simulink model "pservop1"  (Simulink 3.00)
settings: Solver=ode45  StartTime=0.0  StopTime=999999  MaxStep=10  RelTol=1e-3  AbsTol=1e-3
values from neighbouring files (symbols this model uses):
  A1 = 19.63e-4    (= 0.001963)    [pservpar.m]
  A2 = 16.49e-4    (= 0.001649)    [pservpar.m]
  B1 = 30    [pservpar.m]
  Fdry = 0    [pservpar.m]
  g = 9.81    [pservpar.m]
  k1 = 1.4    [pservpar.m]
  kkrit = 1.3154    [pservpar.m]
  kvalve = 2.857e-9    (= 2.857e-09)    [pservpar.m]
  M = 20.    (= 20)    [pservpar.m]
  P10 = 4.e5    (= 400000)    [pservpar.m]
  P20 = (M*g+P10*A1-PR*(A1-A2))/A2    (= 576106.731352)    [pservpar.m]
  PR = 1e5    (= 100000)    [pservpar.m]
  PS = 6e5    (= 600000)    [pservpar.m]
  R1 = 281.3    [pservpar.m]
  rho1 = 1.208    [pservpar.m]
  T1 = 293    [pservpar.m]
  V1 = 4.908e-4    (= 0.0004908)    [pservpar.m]
  V2 = 4.123e-4    (= 0.0004123)    [pservpar.m]
  X0 = 0    [pservpar.m]
  zkrit = 0.528    [pservpar.m]
settings Model: SaveTime=off  SaveOutput=off  Creator=pmn  LastModifiedBy=pmn

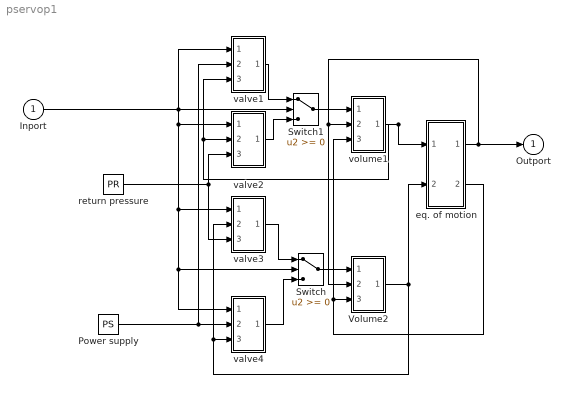
== system pservop1 ==
  Inport : Inport  Port=1  PortWidth=-1  SampleTime=-1  DataType=auto
      settings: SignalType=auto
  Power supply : Constant  Value=PS
  Switch : Switch  Threshold=0
  Switch1 : Switch  Threshold=0
  Volume2 : Subsystem
  eq. of motion : Subsystem
  return pressure : Constant  Value=PR
  valve1 : Subsystem
  valve2 : Subsystem
  valve3 : Subsystem
  valve4 : Subsystem
  volume1 : Subsystem
  Outport : Outport  Port=1
  wires:
  valve3/1(out_1) -> Switch/1
  valve1/1(out_1) -> Switch1/1
  Power supply/1 -> valve4/2(in_2), valve1/2(in_2)
  Inport/1 -> Switch1/2, valve4/1(in_1), Switch/2, valve3/1(in_1), valve2/1(in_1), valve1/1(in_1)
  valve2/1(out_1) -> Switch1/3
  valve4/1(out_1) -> Switch/3
  return pressure/1 -> valve2/3(in_3), valve3/3(in_3)
  volume1/1(out_1) -> eq. of motion/1(in_1), valve2/2(in_2), valve1/3(in_3)
  Switch1/1 -> volume1/1(in_1)
  Switch/1 -> Volume2/1(in_1)
  eq. of motion/1(position) -> Outport/1, Volume2/2(in_2), volume1/2(in_2)
  eq. of motion/2(velocity) -> volume1/3(in_3), Volume2/3(in_3)
  Volume2/1(out_1) -> eq. of motion/2(in_2), valve3/2(in_2), valve4/3(in_3)

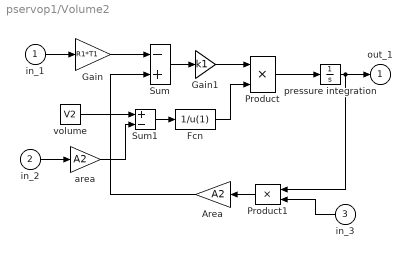
== system pservop1/Volume2 ==
  in_1 : Inport  Port=1  PortWidth=-1  SampleTime=-1  DataType=auto
      settings: SignalType=auto
  in_2 : Inport  Port=2  PortWidth=-1  SampleTime=-1  DataType=auto
      settings: SignalType=auto
  in_3 : Inport  Orientation=left  Port=3  PortWidth=-1  SampleTime=-1  DataType=auto
      settings: SignalType=auto
  Area : Gain  Orientation=left  Gain=A2  SaturateOnIntegerOverflow=on
  Fcn : Fcn  Expr=1/u(1)
  Gain : Gain  Gain=R1*T1  SaturateOnIntegerOverflow=on
  Gain1 : Gain  Gain=k1  SaturateOnIntegerOverflow=on
  Product : Product  Inputs=2  SaturateOnIntegerOverflow=on
  Product1 : Product  Orientation=left  Inputs=2  SaturateOnIntegerOverflow=on
  Sum : Sum  Inputs=-+  SaturateOnIntegerOverflow=on
  Sum1 : Sum  Inputs=+-  SaturateOnIntegerOverflow=on
  area : Gain  Gain=A2  SaturateOnIntegerOverflow=on
  pressure integration : Integrator  ExternalReset=none  InitialConditionSource=internal  InitialCondition=P20  LimitOutput=off  UpperSaturationLimit=inf  LowerSaturationLimit=-inf  ShowSaturationPort=off  ShowStatePort=off  AbsoluteTolerance=auto
  volume : Constant  Value=V2
  out_1 : Outport  Port=1
  wires:
  in_3/1 -> Product1/2
  in_2/1 -> area/1
  in_1/1 -> Gain/1
  Gain/1 -> Sum/1
  volume/1 -> Sum1/1
  Gain1/1 -> Product/1
  Product/1 -> pressure integration/1
  Product1/1 -> Area/1
  Sum/1 -> Gain1/1
  area/1 -> Sum1/2
  Sum1/1 -> Fcn/1
  Fcn/1 -> Product/2
  Area/1 -> Sum/2
  pressure integration/1 -> out_1/1, Product1/1

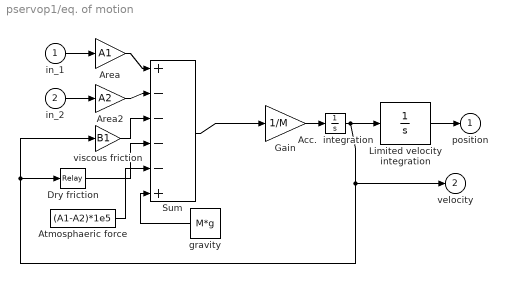
== system pservop1/eq. of motion ==
  in_1 : Inport  Port=1  PortWidth=-1  SampleTime=-1  DataType=auto
      settings: SignalType=auto
  in_2 : Inport  Port=2  PortWidth=-1  SampleTime=-1  DataType=auto
      settings: SignalType=auto
  Acc.  integration : Integrator  ExternalReset=none  InitialConditionSource=internal  InitialCondition=0  LimitOutput=off  UpperSaturationLimit=inf  LowerSaturationLimit=-inf  ShowSaturationPort=off  ShowStatePort=off  AbsoluteTolerance=auto
  Area : Gain  Gain=A1  SaturateOnIntegerOverflow=on
  Area2 : Gain  Gain=A2  SaturateOnIntegerOverflow=on
  Atmosphaeric force : Constant  Value=(A1-A2)*1e5
  Dry friction : Relay  OnSwitchValue=0  OffSwitchValue=0  OnOutputValue=Fdry  OffOutputValue=-Fdry
  Gain : Gain  Gain=1/M  SaturateOnIntegerOverflow=on
  Limited velocity integration : Integrator  ExternalReset=none  InitialConditionSource=internal  InitialCondition=X0  LimitOutput=on  UpperSaturationLimit=0.245  LowerSaturationLimit=-0.245  ShowSaturationPort=off  ShowStatePort=off  AbsoluteTolerance=auto
  Sum : Sum  Inputs=+----+  SaturateOnIntegerOverflow=on
  gravity : Constant  Orientation=left  Value=M*g
  viscous friction : Gain  Gain=B1  SaturateOnIntegerOverflow=on
  position : Outport  Port=1
  velocity : Outport  Port=2
  wires:
  Sum/1 -> Gain/1
  gravity/1 -> Sum/6
  Atmosphaeric force/1 -> Sum/5
  Acc.  integration/1 -> Limited velocity integration/1, velocity/1, viscous friction/1, Dry friction/1
  Limited velocity integration/1 -> position/1
  in_2/1 -> Area2/1
  in_1/1 -> Area/1
  Area/1 -> Sum/1
  Area2/1 -> Sum/2
  viscous friction/1 -> Sum/3
  Gain/1 -> Acc.  integration/1
  Dry friction/1 -> Sum/4

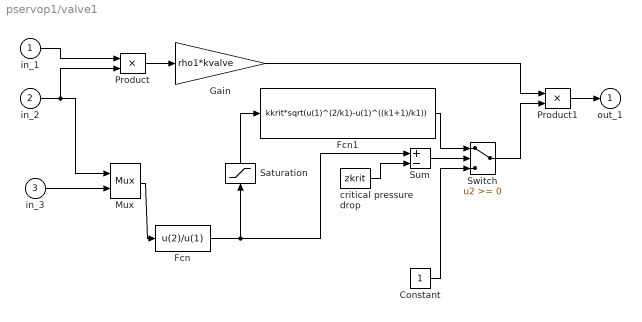
== system pservop1/valve1 ==
  in_1 : Inport  Port=1  PortWidth=-1  SampleTime=-1  DataType=auto
      settings: SignalType=auto
  in_2 : Inport  Port=2  PortWidth=-1  SampleTime=-1  DataType=auto
      settings: SignalType=auto
  in_3 : Inport  Port=3  PortWidth=-1  SampleTime=-1  DataType=auto
      settings: SignalType=auto
  Constant : Constant  Value=1
  Fcn : Fcn  Expr=u(2)/u(1)
  Fcn1 : Fcn  Expr=kkrit*sqrt(u(1)^(2/k1)-u(1)^((k1+1)/k1))
  Gain : Gain  Gain=rho1*kvalve  SaturateOnIntegerOverflow=on
  Mux : Mux  Inputs=2
      settings: DisplayOption=none
  Product : Product  Inputs=2  SaturateOnIntegerOverflow=on
  Product1 : Product  Inputs=2  SaturateOnIntegerOverflow=on
  Saturation : Saturate  Orientation=up  UpperLimit=1  LowerLimit=0
  Sum : Sum  Inputs=+-  SaturateOnIntegerOverflow=on
  Switch : Switch  Threshold=0
  critical pressure drop : Constant  Value=zkrit
  out_1 : Outport  Port=1
  wires:
  in_3/1 -> Mux/2
  Product1/1 -> out_1/1
  in_1/1 -> Product/1
  Product/1 -> Gain/1
  Mux/1 -> Fcn/1
  Constant/1 -> Switch/3
  Sum/1 -> Switch/2
  Fcn1/1 -> Switch/1
  Gain/1 -> Product1/1
  Switch/1 -> Product1/2
  in_2/1 -> Product/2, Mux/1
  critical pressure drop/1 -> Sum/2
  Fcn/1 -> Sum/1, Saturation/1
  Saturation/1 -> Fcn1/1

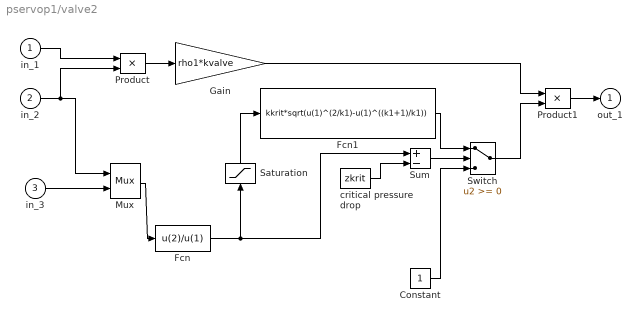
== system pservop1/valve2 ==
  in_1 : Inport  Port=1  PortWidth=-1  SampleTime=-1  DataType=auto
      settings: SignalType=auto
  in_2 : Inport  Port=2  PortWidth=-1  SampleTime=-1  DataType=auto
      settings: SignalType=auto
  in_3 : Inport  Port=3  PortWidth=-1  SampleTime=-1  DataType=auto
      settings: SignalType=auto
  Constant : Constant  Value=1
  Fcn : Fcn  Expr=u(2)/u(1)
  Fcn1 : Fcn  Expr=kkrit*sqrt(u(1)^(2/k1)-u(1)^((k1+1)/k1))
  Gain : Gain  Gain=rho1*kvalve  SaturateOnIntegerOverflow=on
  Mux : Mux  Inputs=2
      settings: DisplayOption=none
  Product : Product  Inputs=2  SaturateOnIntegerOverflow=on
  Product1 : Product  Inputs=2  SaturateOnIntegerOverflow=on
  Saturation : Saturate  Orientation=up  UpperLimit=1  LowerLimit=0
  Sum : Sum  Inputs=+-  SaturateOnIntegerOverflow=on
  Switch : Switch  Threshold=0
  critical pressure drop : Constant  Value=zkrit
  out_1 : Outport  Port=1
  wires:
  in_3/1 -> Mux/2
  Product1/1 -> out_1/1
  in_1/1 -> Product/1
  Product/1 -> Gain/1
  Mux/1 -> Fcn/1
  Constant/1 -> Switch/3
  Sum/1 -> Switch/2
  Fcn1/1 -> Switch/1
  Gain/1 -> Product1/1
  Switch/1 -> Product1/2
  in_2/1 -> Product/2, Mux/1
  critical pressure drop/1 -> Sum/2
  Fcn/1 -> Sum/1, Saturation/1
  Saturation/1 -> Fcn1/1

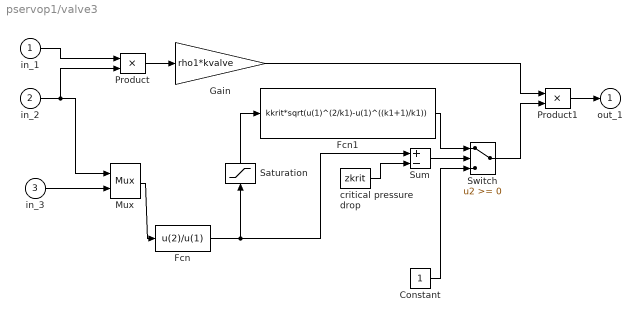
== system pservop1/valve3 ==
  in_1 : Inport  Port=1  PortWidth=-1  SampleTime=-1  DataType=auto
      settings: SignalType=auto
  in_2 : Inport  Port=2  PortWidth=-1  SampleTime=-1  DataType=auto
      settings: SignalType=auto
  in_3 : Inport  Port=3  PortWidth=-1  SampleTime=-1  DataType=auto
      settings: SignalType=auto
  Constant : Constant  Value=1
  Fcn : Fcn  Expr=u(2)/u(1)
  Fcn1 : Fcn  Expr=kkrit*sqrt(u(1)^(2/k1)-u(1)^((k1+1)/k1))
  Gain : Gain  Gain=rho1*kvalve  SaturateOnIntegerOverflow=on
  Mux : Mux  Inputs=2
      settings: DisplayOption=none
  Product : Product  Inputs=2  SaturateOnIntegerOverflow=on
  Product1 : Product  Inputs=2  SaturateOnIntegerOverflow=on
  Saturation : Saturate  Orientation=up  UpperLimit=1  LowerLimit=0
  Sum : Sum  Inputs=+-  SaturateOnIntegerOverflow=on
  Switch : Switch  Threshold=0
  critical pressure drop : Constant  Value=zkrit
  out_1 : Outport  Port=1
  wires:
  in_3/1 -> Mux/2
  Product1/1 -> out_1/1
  in_1/1 -> Product/1
  Product/1 -> Gain/1
  Mux/1 -> Fcn/1
  Constant/1 -> Switch/3
  Sum/1 -> Switch/2
  Fcn1/1 -> Switch/1
  Gain/1 -> Product1/1
  Switch/1 -> Product1/2
  in_2/1 -> Product/2, Mux/1
  critical pressure drop/1 -> Sum/2
  Fcn/1 -> Sum/1, Saturation/1
  Saturation/1 -> Fcn1/1

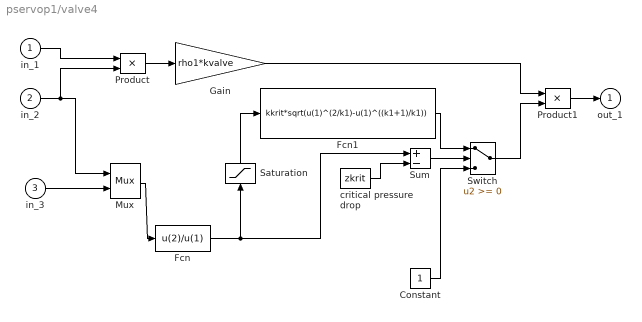
== system pservop1/valve4 ==
  in_1 : Inport  Port=1  PortWidth=-1  SampleTime=-1  DataType=auto
      settings: SignalType=auto
  in_2 : Inport  Port=2  PortWidth=-1  SampleTime=-1  DataType=auto
      settings: SignalType=auto
  in_3 : Inport  Port=3  PortWidth=-1  SampleTime=-1  DataType=auto
      settings: SignalType=auto
  Constant : Constant  Value=1
  Fcn : Fcn  Expr=u(2)/u(1)
  Fcn1 : Fcn  Expr=kkrit*sqrt(u(1)^(2/k1)-u(1)^((k1+1)/k1))
  Gain : Gain  Gain=rho1*kvalve  SaturateOnIntegerOverflow=on
  Mux : Mux  Inputs=2
      settings: DisplayOption=none
  Product : Product  Inputs=2  SaturateOnIntegerOverflow=on
  Product1 : Product  Inputs=2  SaturateOnIntegerOverflow=on
  Saturation : Saturate  Orientation=up  UpperLimit=1  LowerLimit=0
  Sum : Sum  Inputs=+-  SaturateOnIntegerOverflow=on
  Switch : Switch  Threshold=0
  critical pressure drop : Constant  Value=zkrit
  out_1 : Outport  Port=1
  wires:
  in_3/1 -> Mux/2
  Product1/1 -> out_1/1
  in_1/1 -> Product/1
  Product/1 -> Gain/1
  Mux/1 -> Fcn/1
  Constant/1 -> Switch/3
  Sum/1 -> Switch/2
  Fcn1/1 -> Switch/1
  Gain/1 -> Product1/1
  Switch/1 -> Product1/2
  in_2/1 -> Product/2, Mux/1
  critical pressure drop/1 -> Sum/2
  Fcn/1 -> Sum/1, Saturation/1
  Saturation/1 -> Fcn1/1

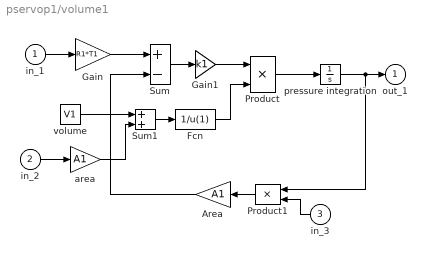
== system pservop1/volume1 ==
  in_1 : Inport  Port=1  PortWidth=-1  SampleTime=-1  DataType=auto
      settings: SignalType=auto
  in_2 : Inport  Port=2  PortWidth=-1  SampleTime=-1  DataType=auto
      settings: SignalType=auto
  in_3 : Inport  Orientation=left  Port=3  PortWidth=-1  SampleTime=-1  DataType=auto
      settings: SignalType=auto
  Area : Gain  Orientation=left  Gain=A1  SaturateOnIntegerOverflow=on
  Fcn : Fcn  Expr=1/u(1)
  Gain : Gain  Gain=R1*T1  SaturateOnIntegerOverflow=on
  Gain1 : Gain  Gain=k1  SaturateOnIntegerOverflow=on
  Product : Product  Inputs=2  SaturateOnIntegerOverflow=on
  Product1 : Product  Orientation=left  Inputs=2  SaturateOnIntegerOverflow=on
  Sum : Sum  Inputs=+-  SaturateOnIntegerOverflow=on
  Sum1 : Sum  Inputs=++  SaturateOnIntegerOverflow=on
  area : Gain  Gain=A1  SaturateOnIntegerOverflow=on
  pressure integration : Integrator  ExternalReset=none  InitialConditionSource=internal  InitialCondition=P10  LimitOutput=off  UpperSaturationLimit=inf  LowerSaturationLimit=-inf  ShowSaturationPort=off  ShowStatePort=off  AbsoluteTolerance=auto
  volume : Constant  Value=V1
  out_1 : Outport  Port=1
  wires:
  pressure integration/1 -> out_1/1, Product1/1
  Area/1 -> Sum/2
  Fcn/1 -> Product/2
  Sum1/1 -> Fcn/1
  area/1 -> Sum1/2
  Sum/1 -> Gain1/1
  Product1/1 -> Area/1
  Product/1 -> pressure integration/1
  Gain1/1 -> Product/1
  volume/1 -> Sum1/1
  Gain/1 -> Sum/1
  in_1/1 -> Gain/1
  in_2/1 -> area/1
  in_3/1 -> Product1/2
